simulink model "case_79_long_full_test"  (R2025b)
settings: Solver=VariableStepAuto  StartTime=0.0  StopTime=850  RelTol=1e-3
settings Model: Creator=sanborkl  LastModifiedBy=admin

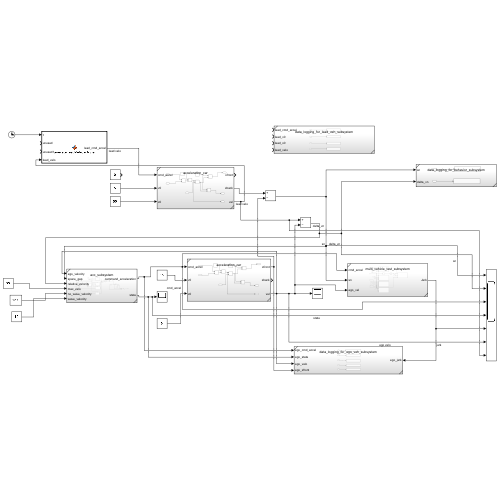
[thumbnail: Simulink's stored preview of the top-level diagram]
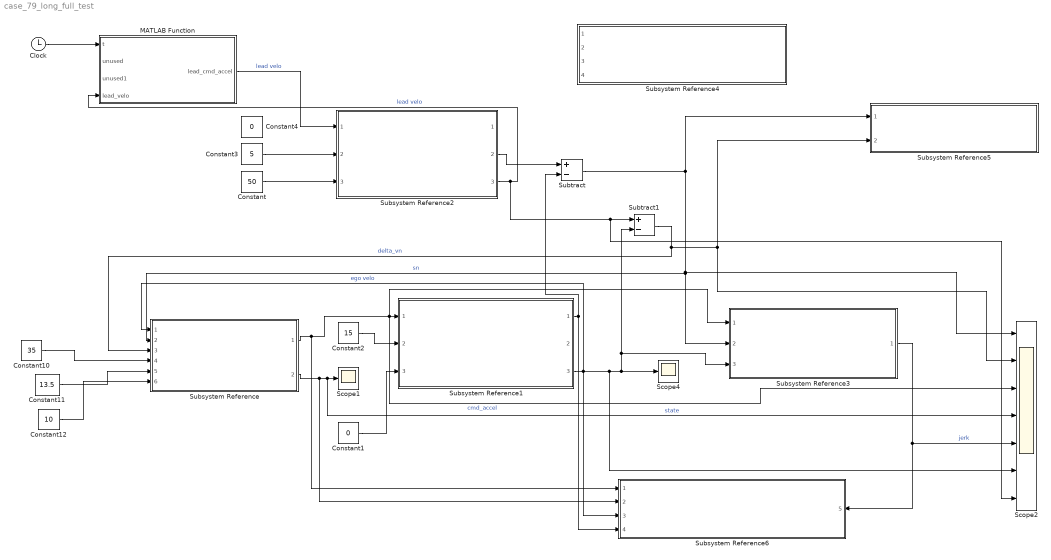
== system case_79_long_full_test ==
  Clock : Clock
  Constant : Constant  Value=50
  Constant1 : Constant  Value=0
  Constant10 : Constant  Value=35
  Constant11 : Constant  Value=13.5
  Constant12 : Constant  Value=10
  Constant2 : Constant  Value=15
  Constant3 : Constant  Value=5
  Constant4 : Constant  Value=0
  MATLAB Function : MATLAB Function  TreatAsAtomicUnit=on
  Scope1 : Scope
      settings: ActiveDisplayYMinimum=-0.24999999999999994  ActiveDisplayYMaximum=2.25  DataLoggingVariableName=ScopeData2
  Scope2 : Scope  NumInputPorts=7
      settings: ActiveDisplayYMinimum=-117.07329181502337  ActiveDisplayYMaximum=307.52238472403315
  Scope4 : Scope
      settings: ActiveDisplayYMinimum=18.125  ActiveDisplayYMaximum=36.875
  Subsystem Reference : Subsystem  ReferencedSubsystem=acc_subsystem
  Subsystem Reference1 : Subsystem  ReferencedSubsystem=acceleration_car
  Subsystem Reference2 : Subsystem  ReferencedSubsystem=acceleration_car
  Subsystem Reference3 : Subsystem  ReferencedSubsystem=multi_vehicle_test_subsystem
  Subsystem Reference4 : Subsystem  ReferencedSubsystem=data_logging_for_lead_veh_subsystem
  Subsystem Reference5 : Subsystem  ReferencedSubsystem=data_logging_for_behavior_subsystem
  Subsystem Reference6 : Subsystem  ReferencedSubsystem=data_logging_for_ego_veh_subsystem
      settings: PortSchema="{\"entries\":[{\"content\":{\"sides\":[{\"content\":{\"connectorIds\":[\"In1\",\"In2\",\"In3\",\"In4\"]},\"type\":\"ConnectorPlacement.EquallySpacedRectSide\",\"uuid\":\"1bb3a8cf-f981-4f8a-aff9-03896ccf7d7c\"},{\"content\":{\"connectorIds\":[\"In5\"],\"side\":\"RIGHT\"},\"type\":\"ConnectorPlacement.EquallySpacedRectSide\",\"uuid\":\"3f6ac5cb-96be-44a3-8993-3635a91bd658\"},{\"content\":{\"side\":\"TOP\"},\"type\":\"ConnectorPlacement.EquallySpacedRectSide\",\"uuid\":\"c641fc7f-a424-4033-b273-2526f6b205c0\"}]},\"type\":\"ConnectorPlacement.EquallySpacedConnector\",\"uuid\":\"2a4be48e-084e-4aa6-b74f-8fe234fedc1a\"}],\"packageUris\":[\"http://schema.mathworks.com/mf0/Connector/R2020b\"],\"version\":\"1.0\"}"
  Subtract : Sum  Inputs=+-
  Subtract1 : Sum  Inputs=+-
  wires:
  Subsystem Reference/1 -> Subsystem Reference6/1, Scope2/3, Subsystem Reference3/1, Subsystem Reference1/1  "cmd_accel"
  Subsystem Reference3/1 -> Subsystem Reference6/5, Scope2/5  "jerk"
  Constant2/1 -> Subsystem Reference1/2
  Constant1/1 -> Subsystem Reference1/3
  Constant3/1 -> Subsystem Reference2/2
  Subsystem Reference1/1 -> Subtract/2, Subsystem Reference6/4
  Subtract1/1 -> Subsystem Reference5/2, Scope2/2, Subsystem Reference/3  "delta_vn"
  Constant/1 -> Subsystem Reference2/3
  Subsystem Reference/2 -> Subsystem Reference6/2, Scope2/4, Scope1/1  "state"
  Subsystem Reference1/3 -> Scope2/6, Subtract1/2, Subsystem Reference3/3, Scope4/1, Subsystem Reference6/3, Subsystem Reference/1  "ego velo"
  Subtract/1 -> Scope2/1, Subsystem Reference3/2, Subsystem Reference/2, Subsystem Reference5/1  "sn"
  Constant12/1 -> Subsystem Reference/6
  Constant10/1 -> Subsystem Reference/4
  Constant11/1 -> Subsystem Reference/5
  Clock/1 -> MATLAB Function/1(t)
  MATLAB Function/1(lead_cmd_accel) -> Subsystem Reference2/1  "lead velo"
  Subsystem Reference2/3 -> Scope2/7, Subtract1/1, MATLAB Function/4(lead_velo)  "lead velo"
  Subsystem Reference2/2 -> Subtract/1

== matlab function case_79_long_full_test/MATLAB Function ==
  data: t input; lead_cmd_accel output; unused input; unused1 input; lead_velo input
function lead_cmd_accel = generateLeadVehicleSignal(t, ~, ~, lead_velo)
    % GENERATELEADVEHICLESIGNAL
    % MATLAB Function for Simulink MATLAB Function block
    % Generates lead vehicle acceleration commands for case_79_long_full_test
    %
    % Inputs:
    %   t          : Current simulation time (seconds)
    %   v_0        : Not used (placeholder for compatibility)
    %   x_0        : Not used (placeholder for compatibility)
    %   lead_velo  : Current lead vehicle velocity (m/s)
    %
    % Output:
    %   lead_cmd_accel : Lead vehicle acceleration command (m/s²)
    %
    % Usage: Place in MATLAB Function block with signature:
    %   lead_cmd_accel = generateLeadVehicleSignal(t, v_0, x_0, lead_velo)
    %
    % Test Timeline (850 seconds):
    %   0-100s    : Mode 0 stable with sinusoidal oscillation (v > 13.5 m/s)
    %   100-200s  : Mode 2 stable with sinusoidal oscillation (v <= 13.5 m/s)
    %   200-400s  : Into wave scenarios (5 x 40s) - decelerate then follow
    %   400-600s  : Out of wave scenarios (5 x 40s) - follow then accelerate
    %   600-750s  : Mode 0 cut-in scenarios (5 x 30s, high-speed)
    %   750-850s  : Mode 2 cut-in scenarios (5 x 20s, low-speed: v <= 13.5 m/s)
    %
    % Mode Classification:
    %   Mode 0: lead_velo > 13.5 m/s (normal highway following)
    %   Mode 2: lead_velo <= 13.5 m/s (urban/low-speed following)

    % =====================================================================
    % SCENARIO 1: Mode 0 Stable Operation (0-100s)
    % Maintain ~25 m/s with sinusoidal oscillation
    % =====================================================================
    if (t > 0) && (t <= 100)
        target_v = 25;

        % Add sinusoidal variation (0.5 Hz, ±3 m/s)
        v_variation = 3 * sin(2*pi*0.5*t);
        desired_v = target_v + v_variation;

        % Simple P-controller: accel = gain * (desired - actual)
        lead_cmd_accel = 0.1 * (desired_v - lead_velo);

        % Limit acceleration
        lead_cmd_accel = max(lead_cmd_accel, -2);
        lead_cmd_accel = min(lead_cmd_accel, 1.5);
        return;
    end

    % =====================================================================
    % SCENARIO 2: Mode 2 Stable Operation (100-200s)
    % Maintain ~10 m/s with sinusoidal oscillation (Mode 2: v <= 13.5 m/s)
    % =====================================================================
    if (t > 100) && (t <= 200)
        target_v = 10;

        % Add sinusoidal variation (0.3 Hz, ±2 m/s)
        t_local = t - 100;
        v_variation = 2 * sin(2*pi*0.3*t_local);
        desired_v = target_v + v_variation;

        lead_cmd_accel = 0.12 * (desired_v - lead_velo);

        % Limit acceleration (Mode 2 is smoother)
        lead_cmd_accel = max(lead_cmd_accel, -1.5);
        lead_cmd_accel = min(lead_cmd_accel, 1.0);
        return;
    end

    % =====================================================================
    % SCENARIOS 3-7: Into Wave (200-400s)
    % Decelerate from Mode 0 (high speed) to Mode 2 (low speed)
    % Crosses Mode threshold at 13.5 m/s
    % 5 scenarios x 40 seconds
    % =====================================================================
    if (t > 200) && (t <= 400)
        t_scenario = t - 200;
        scenario_num = floor(t_scenario / 40) + 1;
        t_local = mod(t_scenario, 40);

        % Each scenario has different initial and target velocities
        initial_vels = [28, 30, 32, 34, 36];  % Mode 0 (>13.5 m/s)
        target_vels = [9, 10, 11, 12, 13];     % Mode 2 (<=13.5 m/s)

        v_initial = initial_vels(scenario_num);
        v_target = target_vels(scenario_num);

        % Smooth deceleration: ramp down over 25 seconds, then oscillate
        if t_local < 25
            % Deceleration phase: linear ramp
            desired_v = v_initial - (v_initial - v_target) * (t_local / 25);
        else
            % Oscillation phase: maintain target with small oscillation
            v_osc = 0.5 * sin(2*pi*0.2*(t_local - 25));
            desired_v = v_target + v_osc;
        end

        lead_cmd_accel = 0.15 * (desired_v - lead_velo);
        lead_cmd_accel = max(lead_cmd_accel, -2.0);
        lead_cmd_accel = min(lead_cmd_accel, 1.0);
        return;
    end

    % =====================================================================
    % SCENARIOS 8-12: Out of Wave (400-600s)
    % Accelerate from Mode 2 (low speed) to Mode 0 (high speed)
    % Crosses Mode threshold at 13.5 m/s
    % 5 scenarios x 40 seconds
    % =====================================================================
    if (t > 400) && (t <= 600)
        t_scenario = t - 400;
        scenario_num = floor(t_scenario / 40) + 1;
        t_local = mod(t_scenario, 40);

        target_vels = [9, 10, 11, 12, 13];     % Mode 2 (<=13.5 m/s)
        final_vels = [28, 30, 32, 34, 36];     % Mode 0 (>13.5 m/s)

        v_target = target_vels(scenario_num);
        v_final = final_vels(scenario_num);

        % Smooth acceleration: oscillate for 15s, then ramp up
        if t_local < 15
            % Initial oscillation phase
            v_osc = 0.3 * sin(2*pi*0.2*t_local);
            desired_v = v_target + v_osc;
        else
            % Acceleration phase: linear ramp
            time_accel = t_local - 15;
            desired_v = v_target + (v_final - v_target) * (time_accel / 25);
        end

        lead_cmd_accel = 0.12 * (desired_v - lead_velo);
        lead_cmd_accel = max(lead_cmd_accel, -1.0);
        lead_cmd_accel = min(lead_cmd_accel, 2.0);
        return;
    end

    % =====================================================================
    % SCENARIOS 13-17: Mode 0 Cut-in Tests (600-750s)
    % Lead vehicle cut-in: sudden appearance, then decelerate to follow
    % 5 scenarios x 30 seconds
    % =====================================================================
    if (t > 600) && (t <= 750)
        t_scenario = t - 600;
        scenario_num = floor(t_scenario / 30) + 1;
        t_local = mod(t_scenario, 30);

        % Parametric cut-in definitions
        ego_vels = [20, 18, 25, 22, 20];
        rel_vels = [10, 15, 20, 15, 10];

        v0 = ego_vels(scenario_num);
        dv = rel_vels(scenario_num);

        cut_in_time = 2;  % Cut-in event at t=2s

        if t_local < cut_in_time
            % Before cut-in: lead is moving faster
            desired_v = v0 + dv;
        else
            % After cut-in: decelerate to ego velocity
            time_since_cut = t_local - cut_in_time;

            if time_since_cut < 8
                % Deceleration phase: ramp down over 8 seconds
                desired_v = (v0 + dv) - dv * (time_since_cut / 8);
            else
                % Settling phase: maintain with slight oscillation
                v_osc = 0.5 * sin(2*pi*0.3*(time_since_cut - 8));
                desired_v = v0 + v_osc;
            end
        end

        % P-controller with physical velocity limit
        lead_cmd_accel = 0.2 * (desired_v - lead_velo);
        lead_cmd_accel = max(lead_cmd_accel, -3.0);
        lead_cmd_accel = min(lead_cmd_accel, 1.5);
        return;
    end

    % =====================================================================
    % SCENARIOS 18-22: Mode 2 Cut-in Tests (750-850s)
    % Low-speed cut-in scenarios
    % 5 scenarios x 20 seconds
    % =====================================================================
    if (t > 750) && (t <= 850)
        t_scenario = t - 750;
        scenario_num = floor(t_scenario / 20) + 1;
        t_local = mod(t_scenario, 20);

        % Mode 2 low-speed cut-in parameters
        ego_vels = [8, 5, 8, 5, 6];
        rel_vels = [5, 5, 5, 5, 4];

        v0 = ego_vels(scenario_num);
        dv = rel_vels(scenario_num);

        cut_in_time = 1;  % Faster cut-in for low speed

        if t_local < cut_in_time
            desired_v = v0 + dv;
        else
            time_since_cut = t_local - cut_in_time;

            if time_since_cut < 5
                % Deceleration phase: ramp down over 5 seconds
                desired_v = (v0 + dv) - dv * (time_since_cut / 5);
            else
                % Settling phase
                v_osc = 0.2 * sin(2*pi*0.2*(time_since_cut - 5));
                desired_v = v0 + v_osc;
            end
        end

        % Mode 2 is smoother with lower acceleration limits
        lead_cmd_accel = 0.15 * (desired_v - lead_velo);
        lead_cmd_accel = max(lead_cmd_accel, -1.5);
        lead_cmd_accel = min(lead_cmd_accel, 1.0);
        return;
    end

    % =====================================================================
    % DEFAULT: Maintain current velocity
    % =====================================================================
    lead_cmd_accel = 0;

end
